simulink model "q_to_l"  (R2018a)
settings: Solver=VariableStepAuto  StartTime=0.0  StopTime=10.0  RelTol=1e-3
settings Model: Creator=MJ  LastModifiedBy=MJ

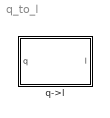
== system q_to_l ==
  q->l : MATLAB Function  TreatAsAtomicUnit=on

== matlab function q_to_l/q->l ==
  data: q input; l output
function l = fcn(q)

q1 = q(1);
q2 = q(2);

l = [sqrt((sin(q1).*(1.0./1.0e1)-3.707106781186548e-1).^2+(cos(q1).*(1.0./1.0e1)-sqrt(2.0).*(1.0./2.0e1)).^2);sqrt((sin(q2).*(1.0./1.0e1)-3.707106781186548e-1).^2+(cos(q2).*(1.0./1.0e1)-sqrt(2.0).*(1.0./2.0e1)).^2)];
